simulink model "rrmc_ol_01"  (R2014a)
settings: Solver=ode1  StartTime=0.0  StopTime=stop_time  FixedStep=step_time  MaxStep=0.01  RelTol=1e-3
values from neighbouring files (symbols this model uses):
  qvet_ini = [-0.0000    1.4526   -2.6861    0.0000    1.2335   -0.0000]    [rrmc_cl_pre_post_01.m]    (also in rrmc_cl_pre_post_01_CopiaProf.m = deg2rad([0 45 -30 -10 -90 -30]); rrmc_ol_pre_post_01.m = [0 0 0 0 30 0]'*pi/180)
  vTCP = [-.5 0 0 1 0 0]'    [rrmc_ol_pre_post_01.m]
libraries: roblocks x2
settings Model: Creator=d029694  LastModifiedBy=Guglielmo
settings DataIOCC: LimitDataPoints=off
settings OptimizationCC: SimCompilerOptimization=off
settings DebuggingCC: MergeDetectMultiDrivingBlocksExec=error  FrameProcessingCompatibilityMsg=error
settings RTWCC: RTWCompilerOptimization=off

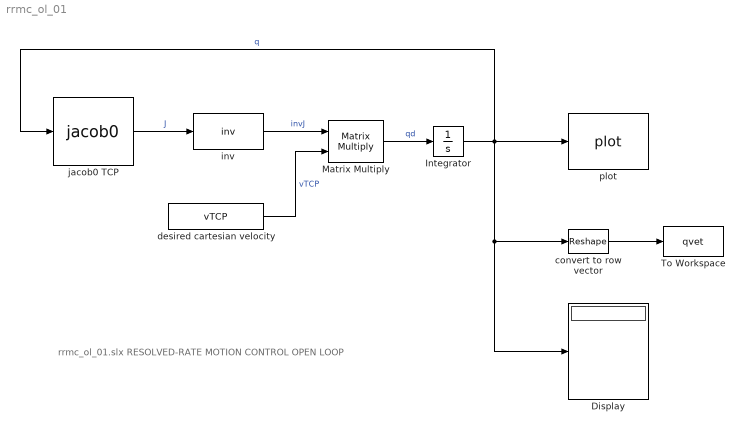
== system rrmc_ol_01 ==
  note: rrmc_ol_01.slx
      |
      | RESOLVED-RATE MOTION CONTROL
      | OPEN LOOP
  Display : Display
  Integrator : Integrator  InitialCondition=qvet_ini
  Matrix Multiply : Product  Multiplication=Matrix(*)
  To Workspace : ToWorkspace  VariableName=qvet  SampleTime=-1
  convert to row vector : Reshape  OutputDimensions=6
  desired cartesian velocity : Constant  Value=vTCP  VectorParams1D=off
  inv : MATLABFcn  MATLABFcn=inv  Output1D=off
  "jacob0 TCP " : roblocks/Kinematics/jacob0   robot=rob6R
  plot : roblocks/Robot Graphics/plot  robot=rob6R  fps=25  holdplot=on
  wires:
  desired cartesian velocity/1 -> Matrix Multiply/2  "vTCP"
  Integrator/1 -> Display/1, convert to row vector/1, "jacob0 TCP "/1, plot/1  "q"
  Matrix Multiply/1 -> Integrator/1  "qd"
  "jacob0 TCP "/1 -> inv/1  "J"
  inv/1 -> Matrix Multiply/1  "invJ"
  convert to row vector/1 -> To Workspace/1
